simulink model "ESP_model"  (R2022b)
settings: Solver=VariableStepAuto  StartTime=0.0  StopTime=tf  MaxStep=1e-3  RelTol=1e-3  EnableMultiTasking=on
undefined symbols (not defined in the file or in its folder): auxdata, magnitude
libraries: slpidlib x1
settings Model: Creator=luca  LastModifiedBy=giacomo
settings SolverCC: AlgebraicLoopSolver=TrustRegion
settings DataIOCC: LimitDataPoints=on  ReturnWorkspaceOutputs=off
settings OptimizationCC: LifeSpan=inf
settings DebuggingCC: UnconnectedInputMsg=warning  UnconnectedOutputMsg=warning  UnconnectedLineMsg=warning  AllowSymbolicDim=off  SFUnexpectedBacktrackingDiag=warning  SFNoUnconditionalDefaultTransitionDiag=warning  SFExecutionAtInitializationDiag=none  SFMachineParentedDataDiag=warning  ArithmeticOperatorsInVariantConditions=warning
settings ModelReferenceCC: EnableRefExpFcnMdlSchedulingChecks=on  PropagateSignalLabelsOutOfModel=off
settings SFSimCC: SimUseLocalCustomCode=off  CustomCodeUndefinedFunction=UseInterfaceOnly
settings RTWCC: RTWUseLocalCustomCode=off
settings CodeAppCC: StateflowObjectComments=on
settings GRTTargetCC: TargetLangStandard=C89/C90 (ANSI)
settings ConfigComp: CovMetricSettings=dw  CovSaveCumulativeToWorkspaceVar=on  CovSaveSingleToWorkspaceVar=on  CovExternalEMLEnable=off

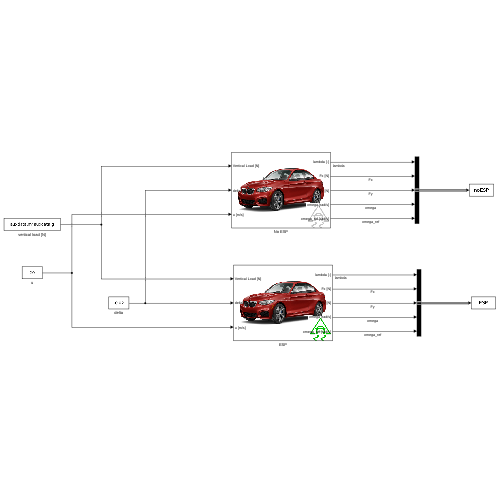
[thumbnail: Simulink's stored preview of the top-level diagram]
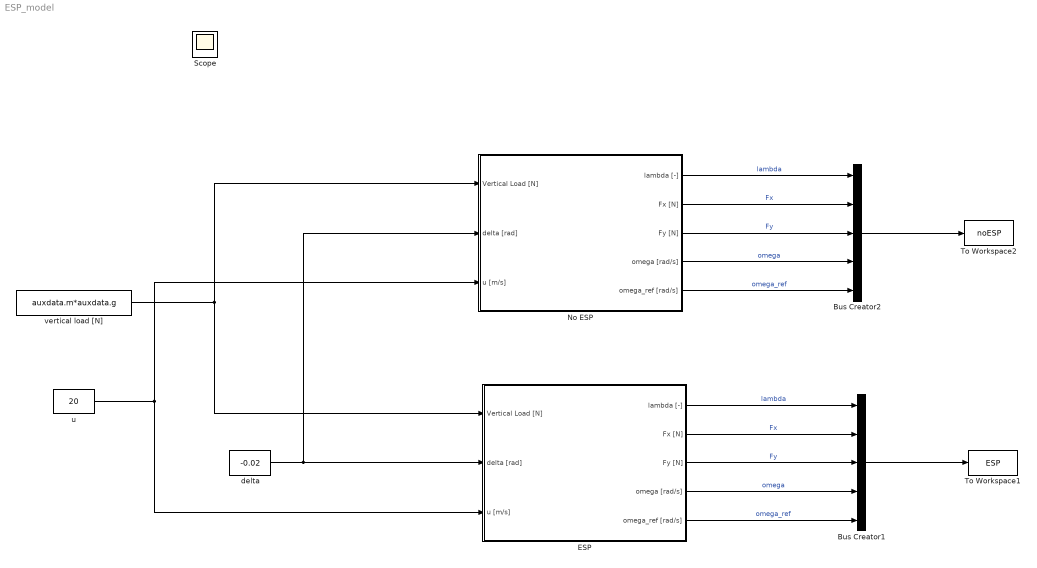
== system ESP_model ==
  Bus Creator1 : BusCreator  Inputs=5
  Bus Creator2 : BusCreator  Inputs=5
  ESP : Subsystem
      mask Display: image('ESPcar_on.png'); % Use "Edit Image" on toolstrip to change.
  No ESP : Subsystem
      mask Display: image('ESPcar_off.png'); % Use "Edit Image" on toolstrip to change.
  To Workspace1 : ToWorkspace  VariableName=ESP  SaveFormat=Timeseries  SampleTime=-1
  To Workspace2 : ToWorkspace  VariableName=noESP  SaveFormat=Timeseries  SampleTime=-1
  delta : Constant  Value=-0.02  SampleTime=-1
  u : Constant  Value=20  SampleTime=-1
  vertical load [N] : Constant  Value=auxdata.m*auxdata.g  SampleTime=-1
  Scope : Scope
  wires:
  vertical load [N]/1 -> No ESP/1(Vertical Load [N]), ESP/1(Vertical Load [N])
  Bus Creator1/1 -> To Workspace1/1
  delta/1 -> No ESP/2(delta [rad]), ESP/2(delta [rad])
  ESP/1(lambda [-]) -> Bus Creator1/1  "lambda"
  ESP/2(" Fx [N]") -> Bus Creator1/2  "Fx"
  ESP/3(" Fy [N]") -> Bus Creator1/3  "Fy"
  ESP/4(" omega [rad/s]") -> Bus Creator1/4  "omega"
  ESP/5(" omega_ref [rad/s]") -> Bus Creator1/5  "omega_ref"
  No ESP/5(" omega_ref [rad/s]") -> Bus Creator2/5  "omega_ref"
  No ESP/1(lambda [-]) -> Bus Creator2/1  "lambda"
  No ESP/4(" omega [rad/s]") -> Bus Creator2/4  "omega"
  No ESP/3(" Fy [N]") -> Bus Creator2/3  "Fy"
  No ESP/2(" Fx [N]") -> Bus Creator2/2  "Fx"
  Bus Creator2/1 -> To Workspace2/1
  u/1 -> ESP/3(u [m/s]), No ESP/3(u [m/s])

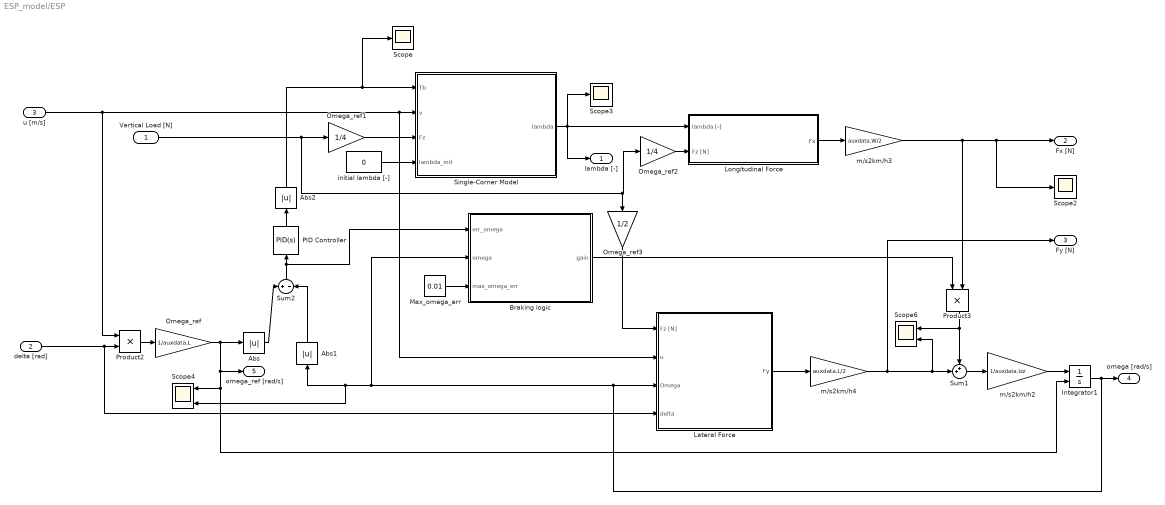
== system ESP_model/ESP ==
  Vertical Load [N] : Inport
  delta [rad] : Inport  Port=2
  u [m/s] : Inport  Port=3
  Abs : Abs  SaturateOnIntegerOverflow=off
  Abs1 : Abs  SaturateOnIntegerOverflow=off
  Abs2 : Abs  SaturateOnIntegerOverflow=off
  Braking logic : Stateflow chart  TreatAsAtomicUnit=on
  Integrator1 : Integrator  InitialConditionSource=external
  Lateral Force : Subsystem
  Longitudinal Force : Subsystem
  Max_omega_err : Constant  Value=0.01
  Omega_ref : Gain  Gain=1/auxdata.L
  Omega_ref1 : Gain  Gain=1/4
  Omega_ref2 : Gain  Gain=1/4
  Omega_ref3 : Gain  Gain=1/2
  PID Controller : slpidlib/PID Controller  Controller=PID  Form=Parallel  TimeDomain=Continuous-time  UseExternalTs=off  SampleTime=-1  IntegratorMethod=Forward Euler  FilterMethod=Forward Euler  ControllerParametersSource=internal  P=10000  I=10000  UseKiTs=off  D=0  N=100  UseFilter=on  TunerSelectOption=Transfer Function Based (PID Tuner App)  InitialConditionSource=internal  InitialConditionForIntegrator=0  InitialConditionForFilter=0  DifferentiatorICPrevScaledInput=0  ExternalReset=none  TrackingMode=off  Kt=1  LimitOutput=off  SatLimitsSource=internal  UpperSaturationLimit=inf  LowerSaturationLimit=-inf  LinearizeAsGain=on  AntiWindupMode=none  Kb=1  LimitIntegrator=off  UpperIntegratorSaturationLimit=inf  LowerIntegratorSaturationLimit=-inf  POutMin=[]  POutMax=[]  IOutMin=[]  IOutMax=[]  DOutMin=[]  DOutMax=[]  NOutMin=[]  NOutMax=[]  SumOutMin=[]  SumOutMax=[]  SaturationOutMin=[]  SaturationOutMax=[]  PParamMin=[]  PParamMax=[]  IParamMin=[]  IParamMax=[]  DParamMin=[]  DParamMax=[]  NParamMin=[]  NParamMax=[]  KbParamMin=[]  KbParamMax=[]  KtParamMin=[]  KtParamMax=[]  KbOutMin=[]  KbOutMax=[]  KtOutMin=[]  KtOutMax=[]  IntegratorOutMin=[]  IntegratorOutMax=[]  FilterOutMin=[]  FilterOutMax=[]  SumI1OutMin=[]  SumI1OutMax=[]  SumI2OutMin=[]  SumI2OutMax=[]  SumI3OutMin=[]  SumI3OutMax=[]  SumI4OutMin=[]  SumI4OutMax=[]  SumDOutMin=[]  SumDOutMax=[]  DifferentiatorOutMin=[]  DifferentiatorOutMax=[]  FilterDiffOutCoefMin=[]  FilterDiffOutCoefMax=[]  ReciprocalOutMin=[]  ReciprocalOutMax=[]  SumDenOutMin=[]  SumDenOutMax=[]  SumNumOutMin=[]  SumNumOutMax=[]  DivideOutMin=[]  DivideOutMax=[]  UdiffTsProdOutMin=[]  UdiffTsProdOutMax=[]  NTsProdOutMin=[]  NTsProdOutMax=[]  UintegralTsProdOutMin=[]  UintegralTsProdOutMax=[]  UngainTsProdOutMin=[]  UngainTsProdOutMax=[]  ClampingZeroOutDataTypeStr=Inherit: Inherit via back propagation  ClampingZeroOutMin=[]  ClampingZeroOutMax=[]  FilterDenConstantOutDataTypeStr=Inherit: Inherit via back propagation  FilterDenConstantOutMin=[]  FilterDenConstantOutMax=[]  PCopyOutDataTypeStr=Inherit: Inherit via back propagation  PCopyOutMin=[]  PCopyOutMax=[]  NCopyOutDataTypeStr=Inherit: Inherit via back propagation  NCopyOutMin=[]  NCopyOutMax=[]  IntegratorContinuousStateAttributes=''  IntegratorStateMustResolveToSignalObject=off  IntegratorRTWStateStorageClass=Auto  FilterContinuousStateAttributes=''  FilterStateMustResolveToSignalObject=off  FilterRTWStateStorageClass=Auto  ParallelPVariant=InternalParameters  IdealPVariant=Disabled  IVariant=InternalParameters  DVariant=InternalParameters  IntegratorVariant=Continuous  SatVariant=Disabled  AWVariant=Passthrough  PCopyVariant=Disabled  TRVariant=Disabled  FdbkBlocksVariant=Forward  IdealPFdbkVariant=Disabled  SatFdbkVariant=Disabled  DerivativeFilterVariant=ContFilter  NVariant=InternalParameters  NCopyVariant=Disabled  FilterICVariant=InternalICsFilter  IntegratorICVariant=InternalICs  ExternalResetVariant=Disabled  TRSumVariant=Passthrough  SumFdbkVariant=Disabled  SumVariant=Sum_PID  TsampFilterVariant=InternalTs  TsampNgainVariant=Passthrough  TsampIntegralVariant=Passthrough  ExternalSaturationOutDataTypeStr=Inherit: Same as second input
  Product2 : Product
  Product3 : Product
  Scope : Scope
  Scope2 : Scope
  Scope3 : Scope
  Scope4 : Scope  NumInputPorts=2
  Scope6 : Scope  NumInputPorts=2
  Single-Corner Model : Subsystem
      mask Display:
      | image('figures/caliper_img.jpeg');
      | color('red');
      | port_label('output',1,'lambda');
      | port_label('input',1,'Tb');
      | port_label('input',2,'v');
      | port_label('input',3,'Fz');
      | port_label('input',4,'lambda_init');
  Sum1 : Sum  Inputs=++|
  Sum2 : Sum  Inputs=+-
  initial lambda [-] : Constant  Value=0
  m/s2km/h2 : Gain  Gain=1/auxdata.Izz
  m/s2km/h3 : Gain  Gain=auxdata.W/2
  m/s2km/h4 : Gain  Gain=auxdata.L/2
  lambda [-] : Outport
  " Fx [N]" : Outport  Port=2
  " Fy [N]" : Outport  Port=3
  " omega [rad/s]" : Outport  Port=4
  " omega_ref [rad/s]" : Outport  Port=5
  wires:
  Single-Corner Model/1(lambda) -> lambda [-]/1, Longitudinal Force/1(lambda [-]), Scope3/1
  Vertical Load [N]/1 -> Omega_ref2/1, Omega_ref3/1, Omega_ref1/1
  initial lambda [-]/1 -> Single-Corner Model/4(lambda_init)
  Longitudinal Force/1(Fx) -> m/s2km/h3/1
  m/s2km/h2/1 -> Integrator1/1
  Integrator1/1 -> Braking logic/2(omega), Abs1/1, Scope4/2, Lateral Force/3(Omega), " omega [rad/s]"/1
  Product2/1 -> Omega_ref/1
  Lateral Force/1(Fy) -> m/s2km/h4/1
  m/s2km/h4/1 -> " Fy [N]"/1, Scope6/2, Sum1/2
  PID Controller/1 -> Abs2/1
  Sum1/1 -> m/s2km/h2/1
  u [m/s]/1 -> Lateral Force/2(u), Single-Corner Model/2(v), Product2/1
  delta [rad]/1 -> Lateral Force/4(delta), Product2/2
  Omega_ref/1 -> Abs/1, " omega_ref [rad/s]"/1, Integrator1/2, Scope4/1
  m/s2km/h3/1 -> Product3/2, " Fx [N]"/1, Scope2/1
  Product3/1 -> Sum1/1, Scope6/1
  Omega_ref1/1 -> Single-Corner Model/3(Fz)
  Omega_ref2/1 -> Longitudinal Force/2(Fz [N])
  Omega_ref3/1 -> Lateral Force/1(Fz [N])
  Braking logic/1(gain) -> Product3/1
  Abs/1 -> Sum2/1
  Abs1/1 -> Sum2/2
  Sum2/1 -> Braking logic/1(err_omega), PID Controller/1
  Abs2/1 -> Scope/1, Single-Corner Model/1(Tb)
  Max_omega_err/1 -> Braking logic/3(max_omega_err)

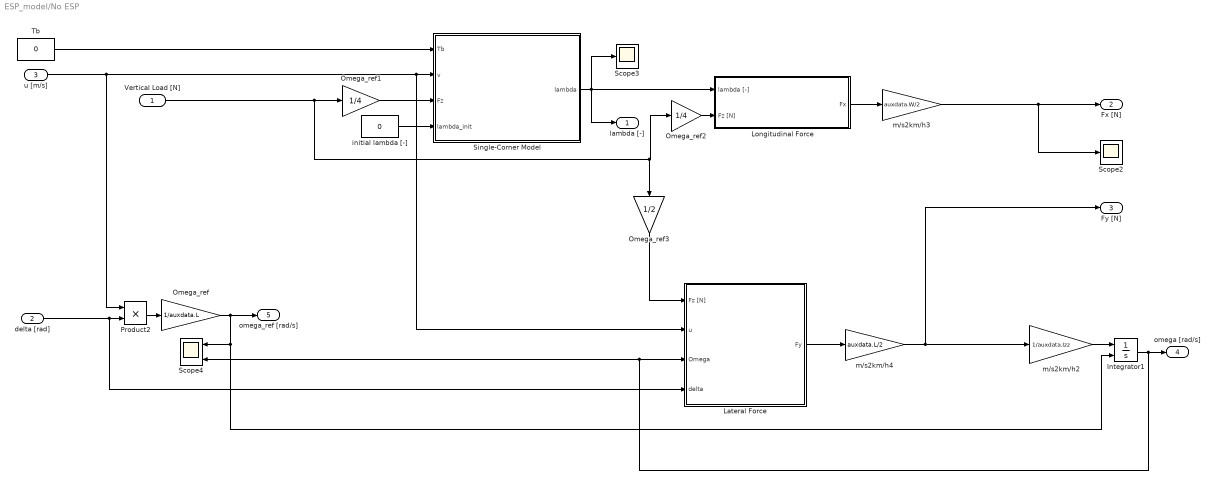
== system ESP_model/No ESP ==
  Vertical Load [N] : Inport
  delta [rad] : Inport  Port=2
  u [m/s] : Inport  Port=3
  Integrator1 : Integrator  InitialConditionSource=external
  Lateral Force : Subsystem
  Longitudinal Force : Subsystem
  Omega_ref : Gain  Gain=1/auxdata.L
  Omega_ref1 : Gain  Gain=1/4
  Omega_ref2 : Gain  Gain=1/4
  Omega_ref3 : Gain  Gain=1/2
  Product2 : Product
  Scope2 : Scope
  Scope3 : Scope
  Scope4 : Scope  NumInputPorts=2
  Single-Corner Model : Subsystem
      mask Display:
      | image('figures/caliper_img.jpeg');
      | color('red');
      | port_label('output',1,'lambda');
      | port_label('input',1,'Tb');
      | port_label('input',2,'v');
      | port_label('input',3,'Fz');
      | port_label('input',4,'lambda_init');
  Tb : Constant  Value=0
  initial lambda [-] : Constant  Value=0
  m/s2km/h2 : Gain  Gain=1/auxdata.Izz
  m/s2km/h3 : Gain  Gain=auxdata.W/2
  m/s2km/h4 : Gain  Gain=auxdata.L/2
  lambda [-] : Outport
  " Fx [N]" : Outport  Port=2
  " Fy [N]" : Outport  Port=3
  " omega [rad/s]" : Outport  Port=4
  " omega_ref [rad/s]" : Outport  Port=5
  wires:
  Single-Corner Model/1(lambda) -> lambda [-]/1, Longitudinal Force/1(lambda [-]), Scope3/1
  Vertical Load [N]/1 -> Omega_ref2/1, Omega_ref3/1, Omega_ref1/1
  initial lambda [-]/1 -> Single-Corner Model/4(lambda_init)
  Longitudinal Force/1(Fx) -> m/s2km/h3/1
  m/s2km/h2/1 -> Integrator1/1
  Integrator1/1 -> Scope4/2, Lateral Force/3(Omega), " omega [rad/s]"/1
  Product2/1 -> Omega_ref/1
  Lateral Force/1(Fy) -> m/s2km/h4/1
  m/s2km/h4/1 -> m/s2km/h2/1, " Fy [N]"/1
  u [m/s]/1 -> Lateral Force/2(u), Single-Corner Model/2(v), Product2/1
  delta [rad]/1 -> Lateral Force/4(delta), Product2/2
  Omega_ref/1 -> Integrator1/2, Scope4/1, " omega_ref [rad/s]"/1
  m/s2km/h3/1 -> " Fx [N]"/1, Scope2/1
  Tb/1 -> Single-Corner Model/1(Tb)
  Omega_ref1/1 -> Single-Corner Model/3(Fz)
  Omega_ref2/1 -> Longitudinal Force/2(Fz [N])
  Omega_ref3/1 -> Lateral Force/1(Fz [N])

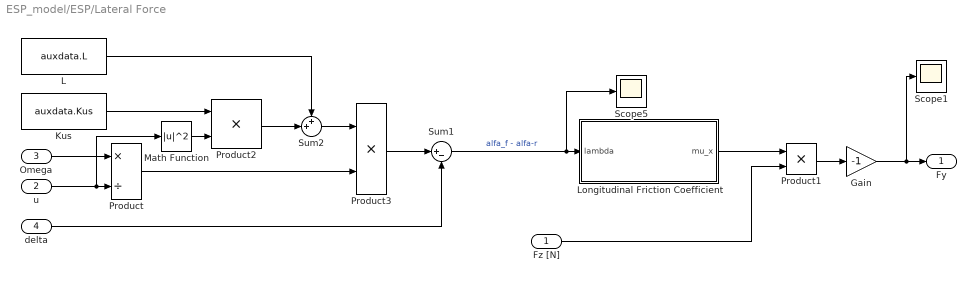
== system ESP_model/ESP/Lateral Force ==
  Fz [N] : Inport
  u : Inport  Port=2
  Omega : Inport  Port=3
  delta : Inport  Port=4
  Gain : Gain  Gain=-1
  Kus : Constant  Value=auxdata.Kus
  L : Constant  Value=auxdata.L
  Longitudinal Friction Coefficient : MATLAB Function  TreatAsAtomicUnit=on
  Math Function : Math  Operator=magnitude^2
  Product : Product  Inputs=*/
  Product1 : Product
  Product2 : Product  Inputs=**
  Product3 : Product  Inputs=**
  Scope1 : Scope
  Scope5 : Scope
  Sum1 : Sum  Inputs=|+-
  Sum2 : Sum  Inputs=++|
  Fy : Outport
  wires:
  u/1 -> Math Function/1, Product/2
  Omega/1 -> Product/1
  Product/1 -> Product3/2
  Gain/1 -> Scope1/1, Fy/1
  Sum1/1 -> Longitudinal Friction Coefficient/1(lambda), Scope5/1  "alfa_f - alfa-r"
  Product1/1 -> Gain/1
  Longitudinal Friction Coefficient/1(mu_x) -> Product1/1
  Fz [N]/1 -> Product1/2
  Kus/1 -> Product2/1
  Math Function/1 -> Product2/2
  Product2/1 -> Sum2/2
  L/1 -> Sum2/1
  delta/1 -> Sum1/2
  Product3/1 -> Sum1/1
  Sum2/1 -> Product3/1

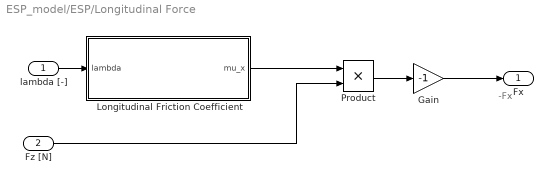
== system ESP_model/ESP/Longitudinal Force ==
  note: -Fx
  lambda [-] : Inport
  Fz [N] : Inport  Port=2
  Gain : Gain  Gain=-1
  Longitudinal Friction Coefficient : MATLAB Function  TreatAsAtomicUnit=on
  Product : Product
  Fx : Outport
  wires:
  Product/1 -> Gain/1
  Gain/1 -> Fx/1
  Longitudinal Friction Coefficient/1(mu_x) -> Product/1
  Fz [N]/1 -> Product/2
  lambda [-]/1 -> Longitudinal Friction Coefficient/1(lambda)

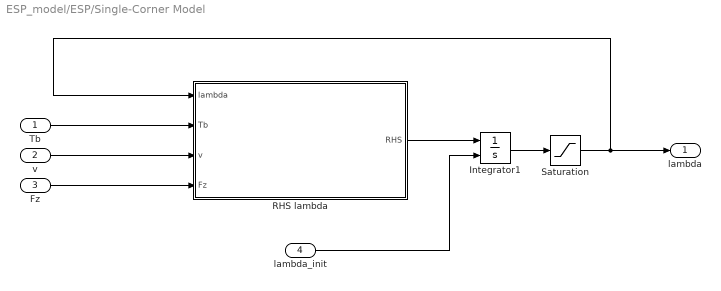
== system ESP_model/ESP/Single-Corner Model ==
  Tb : Inport
  v : Inport  Port=2
  Fz : Inport  Port=3
  lambda_init : Inport  Port=4
  Integrator1 : Integrator  InitialConditionSource=external
  RHS lambda : MATLAB Function  TreatAsAtomicUnit=on
  Saturation : Saturate  UpperLimit=0.99  LowerLimit=0
  lambda : Outport
  wires:
  lambda_init/1 -> Integrator1/2
  RHS lambda/1(RHS) -> Integrator1/1
  v/1 -> RHS lambda/3(v)
  Fz/1 -> RHS lambda/4(Fz)
  Integrator1/1 -> Saturation/1
  Tb/1 -> RHS lambda/2(Tb)
  Saturation/1 -> RHS lambda/1(lambda), lambda/1

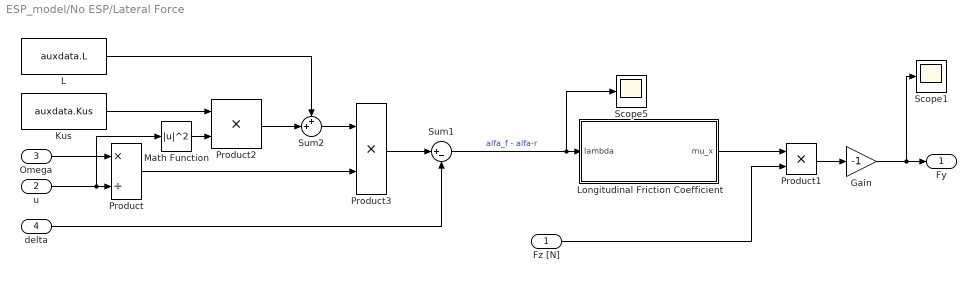
== system ESP_model/No ESP/Lateral Force ==
  Fz [N] : Inport
  u : Inport  Port=2
  Omega : Inport  Port=3
  delta : Inport  Port=4
  Gain : Gain  Gain=-1
  Kus : Constant  Value=auxdata.Kus
  L : Constant  Value=auxdata.L
  Longitudinal Friction Coefficient : MATLAB Function  TreatAsAtomicUnit=on
  Math Function : Math  Operator=magnitude^2
  Product : Product  Inputs=*/
  Product1 : Product
  Product2 : Product  Inputs=**
  Product3 : Product  Inputs=**
  Scope1 : Scope
  Scope5 : Scope
  Sum1 : Sum  Inputs=|+-
  Sum2 : Sum  Inputs=++|
  Fy : Outport
  wires:
  u/1 -> Math Function/1, Product/2
  Omega/1 -> Product/1
  Product/1 -> Product3/2
  Gain/1 -> Scope1/1, Fy/1
  Sum1/1 -> Longitudinal Friction Coefficient/1(lambda), Scope5/1  "alfa_f - alfa-r"
  Product1/1 -> Gain/1
  Longitudinal Friction Coefficient/1(mu_x) -> Product1/1
  Fz [N]/1 -> Product1/2
  Kus/1 -> Product2/1
  Math Function/1 -> Product2/2
  Product2/1 -> Sum2/2
  L/1 -> Sum2/1
  delta/1 -> Sum1/2
  Product3/1 -> Sum1/1
  Sum2/1 -> Product3/1

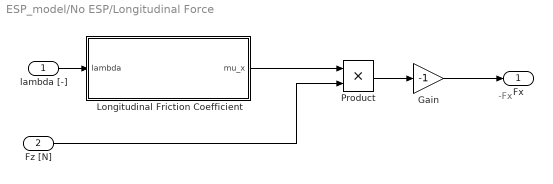
== system ESP_model/No ESP/Longitudinal Force ==
  note: -Fx
  lambda [-] : Inport
  Fz [N] : Inport  Port=2
  Gain : Gain  Gain=-1
  Longitudinal Friction Coefficient : MATLAB Function  TreatAsAtomicUnit=on
  Product : Product
  Fx : Outport
  wires:
  Product/1 -> Gain/1
  Gain/1 -> Fx/1
  Longitudinal Friction Coefficient/1(mu_x) -> Product/1
  Fz [N]/1 -> Product/2
  lambda [-]/1 -> Longitudinal Friction Coefficient/1(lambda)

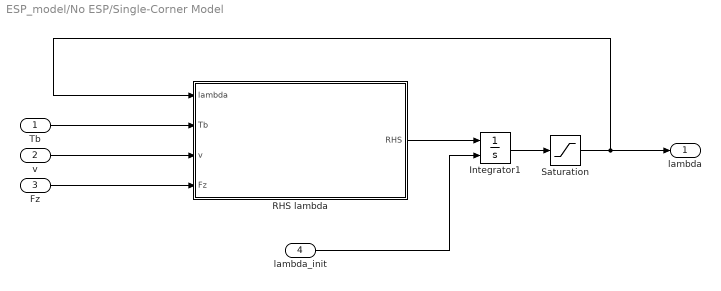
== system ESP_model/No ESP/Single-Corner Model ==
  Tb : Inport
  v : Inport  Port=2
  Fz : Inport  Port=3
  lambda_init : Inport  Port=4
  Integrator1 : Integrator  InitialConditionSource=external
  RHS lambda : MATLAB Function  TreatAsAtomicUnit=on
  Saturation : Saturate  UpperLimit=0.99  LowerLimit=0
  lambda : Outport
  wires:
  lambda_init/1 -> Integrator1/2
  RHS lambda/1(RHS) -> Integrator1/1
  v/1 -> RHS lambda/3(v)
  Fz/1 -> RHS lambda/4(Fz)
  Integrator1/1 -> Saturation/1
  Tb/1 -> RHS lambda/2(Tb)
  Saturation/1 -> RHS lambda/1(lambda), lambda/1

== matlab function ESP_model/No ESP/Longitudinal Force/Longitudinal Friction Coefficient ==
  data: lambda input; mu_x output; auxdata parameter
function mu_x = LongitudinalFrction( lambda, auxdata )
    
mu_x = burckhardt( lambda, auxdata.road_condition );

end

== matlab function ESP_model/No ESP/Single-Corner Model/RHS lambda ==
  data: lambda input; RHS output; Tb input; v input; Fz input; auxdata parameter
function RHS = lambdaDyn( lambda, Tb, v, Fz, auxdata )
% Right hand side of the longitudinal slip dynamics

omega = (1 - lambda) * v / auxdata.r_w;

% Equilibrium manifold
%        /      (1 - lambda) * J \
% Psi = | r_w + ----------------  | * Fz * mu
%        \          r_w * m      /
Psi = (auxdata.r_w + ...
       auxdata.J / (auxdata.r_w * auxdata.m) * (1 - lambda)) * Fz * ...
       burckhardt( lambda, auxdata.road_condition );

if omega <= 0.1
    RHS = 0;
else
    RHS = -(1 - lambda) / (auxdata.J * omega) * (Psi - Tb);
end

end

== matlab function ESP_model/ESP/Lateral Force/Longitudinal Friction Coefficient ==
  data: lambda input; mu_x output; auxdata parameter
function mu_x = LongitudinalFrction( lambda, auxdata )
    
mu_x = burckhardt( lambda, auxdata.road_condition );

end

== stateflow chart ESP_model/ESP/Braking logic ==
  state ESP_ON
    state Brake_front
      state Front_left
        gain = -1;
      state Front_right
        gain = 1;
      (default) -> Front_left
      (junction 30) -> Front_left [order 1] : [omega < 0]
      (junction 30) -> Front_right [order 2] : [omega > 0]
    state Brake_rear
      state Rear_left
        gain = -1;
      state Rear_right
        gain = 1;
      (junction 34) -> Rear_left [order 2] : [omega > 0]
      (junction 34) -> Rear_right [order 1] : [omega < 0]
    (default) -> Brake_front
    Brake_rear -> (junction 25) : [err_omega < 0]
    (junction 25) -> (junction 30) [order 2] : [err_omega < 0]
    (junction 25) -> (junction 34) [order 1] : [err_omega > 0]
    Brake_front -> (junction 25) : [err_omega > 0]
  state ESP_OFF
    gain = 0;
  (default) -> ESP_ON
  ESP_OFF -> (junction 25) : [abs(err_omega) > max_omega_err + 0.01]
  ESP_ON -> ESP_OFF : [abs(err_omega)  < max_omega_err - 0.01]
  data: err_omega input; omega input; max_omega_err input; gain output

== matlab function ESP_model/ESP/Single-Corner Model/RHS lambda ==
  data: lambda input; RHS output; Tb input; v input; Fz input; auxdata parameter
function RHS = lambdaDyn( lambda, Tb, v, Fz, auxdata )
% Right hand side of the longitudinal slip dynamics

omega = (1 - lambda) * v / auxdata.r_w;

% Equilibrium manifold
%        /      (1 - lambda) * J \
% Psi = | r_w + ----------------  | * Fz * mu
%        \          r_w * m      /
Psi = (auxdata.r_w + ...
       auxdata.J / (auxdata.r_w * auxdata.m) * (1 - lambda)) * Fz * ...
       burckhardt( lambda, auxdata.road_condition );

if omega <= 0.1
    RHS = 0;
else
    RHS = -(1 - lambda) / (auxdata.J * omega) * (Psi - Tb);
end

end

== matlab function ESP_model/No ESP/Lateral Force/Longitudinal Friction Coefficient ==
  data: lambda input; mu_x output; auxdata parameter
function mu_x = LongitudinalFrction( lambda, auxdata )
    
mu_x = burckhardt( lambda, auxdata.road_condition );

end

== matlab function ESP_model/ESP/Longitudinal Force/Longitudinal Friction Coefficient ==
  data: lambda input; mu_x output; auxdata parameter
function mu_x = LongitudinalFrction( lambda, auxdata )
    
mu_x = burckhardt( lambda, auxdata.road_condition );

end
